simulink model "zoh"  (R2014b)
settings: Solver=ode45  StartTime=0.0  StopTime=Tend-Ts  RelTol=1e-3
values from neighbouring files (symbols this model uses):
  Ts = 0.00025    [AMB_discrete_parameter.mat]    (also in OKID_AMBsystem_discrete_XY.m = 1e-06; OKID_AMBsystem_discrete_Z.m = 0.01; sys_XY.mat = 1e-06)
settings Model: CovSFcnEnable=on  Creator=BOSS  LastModifiedBy=123
settings OptimizationCC: UseDivisionForNetSlopeComputation=off  SimCompilerOptimization=off
settings DebuggingCC: SolverPrmCheckMsg=none  FrameProcessingCompatibilityMsg=error
settings RTWCC: RTWCompilerOptimization=off

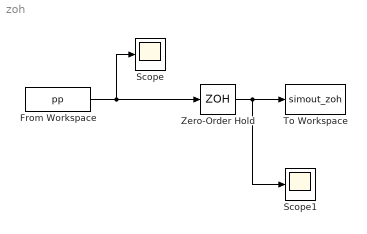
== system zoh ==
  From Workspace : FromWorkspace  VariableName=pp  SampleTime=0
  Scope : Scope
  Scope1 : Scope
  To Workspace : ToWorkspace  VariableName=simout_zoh  SampleTime=-1
  Zero-Order Hold : ZeroOrderHold  SampleTime=Ts
  wires:
  From Workspace/1 -> Scope/1, Zero-Order Hold/1
  Zero-Order Hold/1 -> Scope1/1, To Workspace/1
